simulink model "Test"  (R2018b)
settings: Solver=VariableStepAuto  StartTime=0.0  StopTime=10.0  RelTol=1e-3
undefined symbols (not defined in the file or in its folder): ExpectedOutputs, Inputs, sigbuilder_block, TestCase, TestInps, TestIters
libraries: fillib x3, library x2
(part 1 of 7)
settings Model: Creator=gauthamsm  LastModifiedBy=gauthamsm

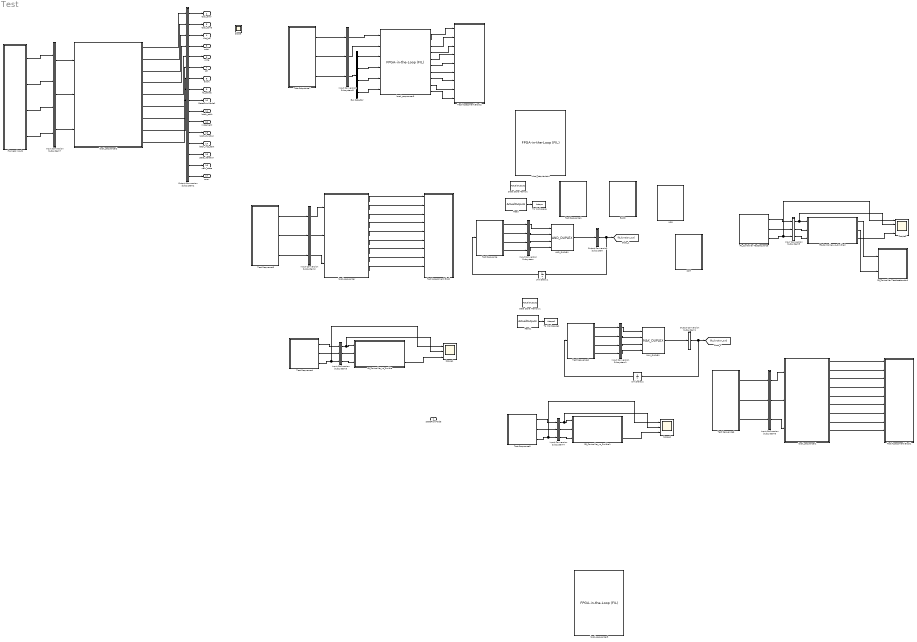
== system Test ==
  " XOR" : Test Sequence  TreatAsAtomicUnit=on
  AND_DUPLEX : library/AND_DUPLEX  SystemSampleTime=-1  VariantControl=MUX_FB
  BAND : Test Sequence  TreatAsAtomicUnit=on
  Bus Selector : BusSelector  OutputSignals=done,busy,error,code
  Data Store Memory : DataStoreMemory  DataStoreName=ActualOutputs  ReadBeforeWriteMsg=warning  WriteAfterWriteMsg=warning  WriteAfterReadMsg=warning  ShowAdditionalParam=off  OutDataTypeStr=int32  Dimensions=[TestIters, 3]
  Data Store Memory1 : DataStoreMemory  DataStoreName=ActualOutputs  ReadBeforeWriteMsg=warning  WriteAfterWriteMsg=warning  WriteAfterReadMsg=warning  ShowAdditionalParam=off  OutDataTypeStr=int32  Dimensions=[TestIters, 3]
  FB_Controller_vs_Smitha : ModelReference  ModelNameDialog=FB_Controller_vs_Smitha  SimulationMode=Normal  ModelReferenceVersion=1.41
  FB_Controller_vs_Smitha1 : ModelReference  ModelNameDialog=FB_Controller_vs_Smitha  SimulationMode=Normal  ModelReferenceVersion=1.41
  FB_Controller_vs_Smitha2 : ModelReference  ModelNameDialog=FB_Controller  SimulationMode=Normal  ModelReferenceVersion=1.46
  Fb_Controller TestAssessment : Test Sequence  TreatAsAtomicUnit=on
  Fb_Controller TestSequence : Test Sequence  TreatAsAtomicUnit=on
  Harness Inputs : Subsystem  Tag=STV Subsys  LoadFcn=sigbuilder_block('load');  StartFcn=sigbuilder_block('start');  StopFcn=sigbuilder_block('stop');  ClipboardFcn=sigbuilder_block('clipboard');  mask(Sigbuilder block){tuvar=[0:10]}
      mask init:
      | if ~strcmp(get_param(bdroot(gcb),'SimulationStatus'),'stopped'),tuvar = sigbuilder_block('maskInit'); end
      settings: CopyFcn=sigbuilder_block('copy');  DeleteFcn=sigbuilder_block('delete');  ModelCloseFcn=sigbuilder_block('modelClose');  PreSaveFcn=sigbuilder_block('preSave');  PauseFcn=sigbuilder_block('pause');  ContinueFcn=sigbuilder_block('continue');  NameChangeFcn=sigbuilder_block('namechange');  OpenFcn=sigbuilder_block('open',[5.4 30 1141.2 522.6 ]);  CloseFcn=sigbuilder_block('close');
      mask Display: plot(0, 0, 100, 100,[2, 2, 32, 32, 2], [68, 8, 8, 68, 68],[32, 2], [38, 38], [32, 19, 2],[53, 60, 44], [32, 17, 17, 2],[16, 16, 31, 31]);txt = getActiveGroup(gcbh);text(2, 100, txt,'verticalAlignment', 'top');
  Input Conversion Subsystem : Subsystem  Tag=__SLT_ICS__  Description=|
      | Signal spec.
      | and routing
      settings: AttributesFormatString=%<Description>
  Input Conversion Subsystem1 : Subsystem  Tag=__SLT_ICS__  Description=|
      | Signal spec.
      | and routing
      settings: AttributesFormatString=%<Description>
  Input Conversion Subsystem2 : Subsystem  Tag=__SLT_ICS__  Description=|
      | Signal spec.
      | and routing
      settings: AttributesFormatString=%<Description>
  Input Conversion Subsystem3 : Subsystem  Tag=__SLT_ICS__  Description=|
      | Signal spec.
      | and routing
      settings: AttributesFormatString=%<Description>
  Input Conversion Subsystem4 : Subsystem  Tag=__SLT_ICS__  Description=|
      | Signal spec.
      | and routing
      settings: AttributesFormatString=%<Description>
  Input Conversion Subsystem5 : Subsystem  Tag=__SLT_ICS__  Description=|
      | Signal spec.
      | and routing
      settings: AttributesFormatString=%<Description>
  Input Conversion Subsystem6 : Subsystem  Tag=__SLT_ICS__  Description=|
      | Signal spec.
      | and routing
      settings: AttributesFormatString=%<Description>
  Input Conversion Subsystem7 : Subsystem  Tag=__SLT_ICS__  Description=|
      | Signal spec.
      | and routing
      settings: AttributesFormatString=%<Description>
  Input Conversion Subsystem8 : Subsystem  Tag=__SLT_ICS__  Description=|
      | Signal spec.
      | and routing
      settings: AttributesFormatString=%<Description>
  MAX_DUPLEX : library/MAX_DUPLEX  SystemSampleTime=-1  VariantControl=MUX_FB
  NOT : Test Sequence  TreatAsAtomicUnit=on
  Output Conversion Subsystem : Subsystem  Tag=__SLT_OCS__  Description=|
      | Signal spec.
      | and routing
      settings: AttributesFormatString=%<Description>
  Output Conversion Subsystem1 : Subsystem  Tag=__SLT_OCS__  Description=|
      | Signal spec.
      | and routing
      settings: AttributesFormatString=%<Description>
  Output Conversion Subsystem2 : Subsystem  Tag=__SLT_OCS__  Description=|
      | Signal spec.
      | and routing
      settings: AttributesFormatString=%<Description>
  Read : DataStoreRead  DataStoreName=ActualOutputs
  Read1 : DataStoreRead  DataStoreName=ActualOutputs
  Scope : Scope
  Scope1 : Scope  NumInputPorts=3
  Scope2 : Scope  NumInputPorts=3
  Scope3 : Scope  NumInputPorts=4
  Test Assessment Block : Test Sequence  Tag=__SLT_ASMT__  TreatAsAtomicUnit=on
  Test Assessment Block1 : Test Sequence  Tag=__SLT_ASMT__  TreatAsAtomicUnit=on
  Test Assessment Block2 : Test Sequence  Tag=__SLT_ASMT__  TreatAsAtomicUnit=on
  Test Sequence : Test Sequence  TreatAsAtomicUnit=on
  Test Sequence1 : Test Sequence  TreatAsAtomicUnit=on
  Test Sequence2 : Test Sequence  TreatAsAtomicUnit=on
  Test Sequence3 : Test Sequence  TreatAsAtomicUnit=on
  Test Sequence4 : Test Sequence  TreatAsAtomicUnit=on
  Test Sequence5 : Test Sequence  TreatAsAtomicUnit=on
  Test Sequence6 : Test Sequence  TreatAsAtomicUnit=on
  Test Sequence7 : Test Sequence  TreatAsAtomicUnit=on
  To Workspace : ToWorkspace  VariableName=Actops  SampleTime=-1
  To Workspace1 : ToWorkspace  VariableName=Actops1  SampleTime=-1
  Unit Delay1 : UnitDelay  SampleTime=-1
  Unit Delay2 : UnitDelay  SampleTime=-1
  local_sequencer : ModelReference  ModelNameDialog=local_sequencer  SimulationMode=Normal  ModelReferenceVersion=1.256
  local_sequencer1 : ModelReference  ModelNameDialog=local_sequencer  SimulationMode=Normal  ModelReferenceVersion=1.256
  local_sequencer2 : ModelReference  ModelNameDialog=local_sequencer  SimulationMode=Normal  ModelReferenceVersion=1.256
  local_sequencer3 : fillib/FPGA-in-the-Loop (FIL)  ForceInterfaceUpdate=0.81472
  local_sequencer4 : fillib/FPGA-in-the-Loop (FIL)  ForceInterfaceUpdate=0.90579
  local_sequencer5 : fillib/FPGA-in-the-Loop (FIL)  ForceInterfaceUpdate=0.91338
  StateFlowMode : Outport
  task_error : Outport  Port=2  OutDataTypeStr=boolean  PortDimensions=[1]
  task_done : Outport  Port=3  OutDataTypeStr=boolean  PortDimensions=[1]
  inst_ptr : Outport  Port=4  OutDataTypeStr=uint32  PortDimensions=[1]
  addr : Outport  Port=5  OutDataTypeStr=fixdt('ufix8_En1000')  PortDimensions=[1]
  write : Outport  Port=6  OutDataTypeStr=boolean  PortDimensions=[1]
  ctrl : Outport  Port=7  OutDataTypeStr=boolean  PortDimensions=[1]
  abort : Outport  Port=8  OutDataTypeStr=boolean  PortDimensions=[1]
  fb_select : Outport  Port=9  OutDataTypeStr=uint8  PortDimensions=[1]
  StateFlowMode1 : Outport  Port=10  OutDataTypeStr=Enum: StateFlowModeType  PortDimensions=[1]
  latch_addr : Outport  Port=11  OutDataTypeStr=boolean  PortDimensions=[1]
  increment : Outport  Port=12  OutDataTypeStr=boolean  PortDimensions=[1]
  latch_function : Outport  Port=13  OutDataTypeStr=boolean  PortDimensions=[1]
  latch_inst_start : Outport  Port=14  OutDataTypeStr=boolean  PortDimensions=[1]
  state_iteration : Outport  Port=15  OutDataTypeStr=boolean  PortDimensions=[1]
  new_state : Outport  Port=16  OutDataTypeStr=boolean  PortDimensions=[1]
  error : Outport  Port=17  OutDataTypeStr=boolean  PortDimensions=[1]
  wires:
  Unit Delay1/1 -> Test Sequence/1(fb_functions_out)
  Output Conversion Subsystem/1(Outport_1) -> Unit Delay1/1, [fb_function_out]
  Input Conversion Subsystem/3(Outport_3) -> AND_DUPLEX/3
  AND_DUPLEX/1 -> Output Conversion Subsystem/1(Inport_1)
  Input Conversion Subsystem/4(Outport_4) -> AND_DUPLEX/4
  Test Sequence/2(fb_control) -> Input Conversion Subsystem/2(Inport_2)
  Input Conversion Subsystem/1(Outport_1) -> AND_DUPLEX/1
  Input Conversion Subsystem/2(Outport_2) -> AND_DUPLEX/2
  Test Sequence/3(dataInA) -> Input Conversion Subsystem/3(Inport_3)
  Test Sequence/4(dataInB) -> Input Conversion Subsystem/4(Inport_4)
  Test Sequence/1(fb_select) -> Input Conversion Subsystem/1(Inport_1)
  Read/1 -> To Workspace/1
  Input Conversion Subsystem1/3(Outport_3) -> MAX_DUPLEX/3
  Test Sequence2/4(dataInB) -> Input Conversion Subsystem1/4(Inport_4)
  Input Conversion Subsystem1/4(Outport_4) -> MAX_DUPLEX/4
  Unit Delay2/1 -> Test Sequence2/1(fb_functions_out)
  Output Conversion Subsystem1/1(Outport_1) -> Unit Delay2/1, [fb_function_out]
  Read1/1 -> To Workspace1/1
  Test Sequence2/1(fb_select) -> Input Conversion Subsystem1/1(Inport_1)
  Input Conversion Subsystem1/1(Outport_1) -> MAX_DUPLEX/1
  Input Conversion Subsystem1/2(Outport_2) -> MAX_DUPLEX/2
  MAX_DUPLEX/1 -> Output Conversion Subsystem1/1(Inport_1)
  Test Sequence2/2(fb_control) -> Input Conversion Subsystem1/2(Inport_2)
  Test Sequence2/3(dataInA) -> Input Conversion Subsystem1/3(Inport_3)
  Test Sequence3/2(inst) -> Input Conversion Subsystem2/2(Inport_2)
  local_sequencer/2 -> Test Assessment Block/2(task_done)  "task_done"
  local_sequencer/8 -> Test Assessment Block/8(fb_select)  "fb_select"
  ? -> Test Assessment Block/10(latch_addr)  "latch_addr"
  Input Conversion Subsystem2/1(Outport_1) -> local_sequencer/1
  Test Sequence3/1(trigger) -> Input Conversion Subsystem2/1(Inport_1)
  local_sequencer/3 -> Test Assessment Block/3(inst_ptr)  "inst_ptr"
  Input Conversion Subsystem2/3(Outport_3) -> local_sequencer/3
  Input Conversion Subsystem2/2(Outport_2) -> local_sequencer/2
  local_sequencer/1 -> Test Assessment Block/1(task_error)  "task_error"
  local_sequencer/7 -> Test Assessment Block/7(abort)  "abort"
  local_sequencer/6 -> Test Assessment Block/6(ctrl)  "ctrl"
  local_sequencer/9 -> Test Assessment Block/9(StateFlowMode)  "StateFlowMode"
  local_sequencer/5 -> Test Assessment Block/5(write)  "write"
  local_sequencer/4 -> Test Assessment Block/4(addr)  "addr"
  Test Sequence3/3(status) -> Input Conversion Subsystem2/3(Inport_3)
  Test Sequence4/3(fb_func_signals) -> Scope1/1, Input Conversion Subsystem3/3(Inport_3)
  Input Conversion Subsystem3/3(Outport_3) -> FB_Controller_vs_Smitha/3
  Test Sequence4/1(ctrl) -> Input Conversion Subsystem3/1(Inport_1)
  Input Conversion Subsystem3/1(Outport_1) -> Scope1/2, FB_Controller_vs_Smitha/1
  Test Sequence4/2(abort) -> Input Conversion Subsystem3/2(Inport_2)
  FB_Controller_vs_Smitha/3 -> Scope1/3
  Input Conversion Subsystem3/2(Outport_2) -> FB_Controller_vs_Smitha/2
  FB_Controller_vs_Smitha1/3 -> Scope2/3
  Input Conversion Subsystem4/1(Outport_1) -> Scope2/2, FB_Controller_vs_Smitha1/1
  Input Conversion Subsystem4/2(Outport_2) -> FB_Controller_vs_Smitha1/2
  Input Conversion Subsystem4/3(Outport_3) -> FB_Controller_vs_Smitha1/3
  Test Sequence5/3(fb_func_signals) -> Scope2/1, Input Conversion Subsystem4/3(Inport_3)
  Test Sequence5/2(abort) -> Input Conversion Subsystem4/2(Inport_2)
  Test Sequence5/1(ctrl) -> Input Conversion Subsystem4/1(Inport_1)
  Fb_Controller TestSequence/3(fb_func_signals) -> Scope3/1, Input Conversion Subsystem5/3(Inport_3)
  Fb_Controller TestSequence/2(abort) -> Input Conversion Subsystem5/2(Inport_2)
  Input Conversion Subsystem5/2(Outport_2) -> FB_Controller_vs_Smitha2/2
  FB_Controller_vs_Smitha2/3 -> Scope3/4
  FB_Controller_vs_Smitha2/2 -> Fb_Controller TestAssessment/2(status)
  FB_Controller_vs_Smitha2/1 -> Fb_Controller TestAssessment/1(fb_control)
  Fb_Controller TestSequence/1(ctrl) -> Input Conversion Subsystem5/1(Inport_1)
  Input Conversion Subsystem5/1(Outport_1) -> Scope3/2, FB_Controller_vs_Smitha2/1
  Input Conversion Subsystem5/3(Outport_3) -> FB_Controller_vs_Smitha2/3
  local_sequencer1/5 -> Test Assessment Block1/5(write)  "write"
  ? -> Test Assessment Block1/10(latch_addr)  "latch_addr"
  local_sequencer1/9 -> Test Assessment Block1/9(StateFlowMode)  "StateFlowMode"
  local_sequencer1/6 -> Test Assessment Block1/6(ctrl)  "ctrl"
  local_sequencer1/7 -> Test Assessment Block1/7(abort)  "abort"
  local_sequencer1/8 -> Test Assessment Block1/8(fb_select)  "fb_select"
  local_sequencer1/3 -> Test Assessment Block1/3(inst_ptr)  "inst_ptr"
  Test Sequence6/1(trigger) -> Input Conversion Subsystem6/1(Inport_1)
  local_sequencer1/4 -> Test Assessment Block1/4(addr)  "addr"
  Test Sequence6/2(inst) -> Input Conversion Subsystem6/2(Inport_2)
  local_sequencer1/1 -> Test Assessment Block1/1(task_error)  "task_error"
  local_sequencer1/2 -> Test Assessment Block1/2(task_done)  "task_done"
  Input Conversion Subsystem6/3(Outport_3) -> local_sequencer1/3
  Test Sequence6/3(status) -> Input Conversion Subsystem6/3(Inport_3)
  Input Conversion Subsystem6/2(Outport_2) -> local_sequencer1/2
  Input Conversion Subsystem6/1(Outport_1) -> local_sequencer1/1
  Output Conversion Subsystem2/6(Outport_6) -> ctrl/1
  Output Conversion Subsystem2/3(Outport_3) -> inst_ptr/1
  ? -> Output Conversion Subsystem2/13(Inport_13)
  local_sequencer2/5 -> Output Conversion Subsystem2/5(Inport_5)
  local_sequencer2/9 -> Output Conversion Subsystem2/9(Inport_9)
  Input Conversion Subsystem7/3(Outport_3) -> local_sequencer2/3
  Output Conversion Subsystem2/16(Outport_16) -> error/1
  ? -> Output Conversion Subsystem2/10(Inport_10)
  Input Conversion Subsystem7/1(Outport_1) -> local_sequencer2/1
  local_sequencer2/7 -> Output Conversion Subsystem2/7(Inport_7)
  Output Conversion Subsystem2/13(Outport_13) -> latch_inst_start/1
  local_sequencer2/6 -> Output Conversion Subsystem2/6(Inport_6)
  Output Conversion Subsystem2/9(Outport_9) -> StateFlowMode1/1
  Output Conversion Subsystem2/11(Outport_11) -> increment/1
  local_sequencer2/3 -> Output Conversion Subsystem2/3(Inport_3)
  local_sequencer2/1 -> Output Conversion Subsystem2/1(Inport_1)
  Output Conversion Subsystem2/14(Outport_14) -> state_iteration/1
  local_sequencer2/8 -> Output Conversion Subsystem2/8(Inport_8)
  Output Conversion Subsystem2/15(Outport_15) -> new_state/1
  Input Conversion Subsystem7/2(Outport_2) -> local_sequencer2/2
  local_sequencer2/2 -> Output Conversion Subsystem2/2(Inport_2)
  Harness Inputs/4(status.code) -> Input Conversion Subsystem7/4(Inport_4)
  ? -> Output Conversion Subsystem2/14(Inport_14)
  Output Conversion Subsystem2/5(Outport_5) -> write/1
  local_sequencer2/4 -> Output Conversion Subsystem2/4(Inport_4)
  ? -> Output Conversion Subsystem2/16(Inport_16)
  Harness Inputs/2(inst) -> Input Conversion Subsystem7/2(Inport_2)
  Output Conversion Subsystem2/2(Outport_2) -> task_done/1
  ? -> Output Conversion Subsystem2/12(Inport_12)
  Output Conversion Subsystem2/1(Outport_1) -> task_error/1
  Output Conversion Subsystem2/8(Outport_8) -> fb_select/1
  Harness Inputs/1(trigger) -> Input Conversion Subsystem7/1(Inport_1)
  Output Conversion Subsystem2/7(Outport_7) -> abort/1
  Output Conversion Subsystem2/10(Outport_10) -> latch_addr/1
  Output Conversion Subsystem2/12(Outport_12) -> latch_function/1
  ? -> Output Conversion Subsystem2/15(Inport_15)
  Harness Inputs/3(status.error) -> Input Conversion Subsystem7/3(Inport_3)
  ? -> Output Conversion Subsystem2/11(Inport_11)
  Output Conversion Subsystem2/4(Outport_4) -> addr/1
  Bus Selector/4 -> local_sequencer5/6  "<code>"
  Test Sequence7/3(status) -> Input Conversion Subsystem8/3(Inport_3)
  Test Sequence7/1(trigger) -> Input Conversion Subsystem8/1(Inport_1)
  Input Conversion Subsystem8/1(Outport_1) -> local_sequencer5/1
  Test Sequence7/2(inst) -> Input Conversion Subsystem8/2(Inport_2)
  local_sequencer5/10 -> Test Assessment Block2/9(latch_addr)
  Bus Selector/2 -> local_sequencer5/4  "<busy>"
  local_sequencer5/5 -> Test Assessment Block2/4(addr)
  local_sequencer5/8 -> Test Assessment Block2/7(abort)
  local_sequencer5/3 -> Test Assessment Block2/2(task_done)
  local_sequencer5/6 -> Test Assessment Block2/5(write)
  local_sequencer5/2 -> Test Assessment Block2/1(task_error)
  local_sequencer5/4 -> Test Assessment Block2/3(inst_ptr)
  Input Conversion Subsystem8/2(Outport_2) -> local_sequencer5/2
  Bus Selector/1 -> local_sequencer5/3  "<done>"
  local_sequencer5/7 -> Test Assessment Block2/6(ctrl)
  Bus Selector/3 -> local_sequencer5/5  "<error>"
  Input Conversion Subsystem8/3(Outport_3) -> Bus Selector/1
  local_sequencer5/9 -> Test Assessment Block2/8(fb_select)

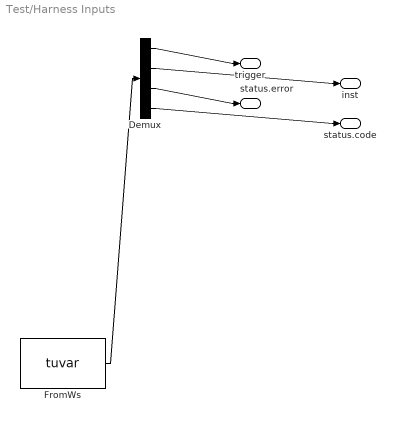
== system Test/Harness Inputs ==
  Demux : Demux  Tag=STV Demux
  FromWs : FromWorkspace  Tag=STV FromWs  VariableName=tuvar  SampleTime=0
      SigBuilderData=|
      | dataSet(1).timeRange = [0 6]
      | dataSet(1).name = 'Test Case 1'
      | dataSet(2).timeRange = [0 7]
      | dataSet(2).name = 'Test Case 2'
      | dataSet(3).timeRange = [0 8]
      | dataSet(3).name = 'Test Case 3'
      | dataSet(4).timeRange = [0 9]
      | dataSet(4).name = 'Test Case 4'
      | dataSet(5).timeRange = [0 10]
      | dataSet(5).name = 'Test Case 5'
      | dataSet(6).timeRange = [0 12]
      | dataSet(6).name = 'Test Case 6'
      | dataSet(7).timeRange = [0 14]
      | dataSet(7).name = 'Test Case 7'
      | dataSet(8).timeRange = [0 15]
      | dataSet(8).name = 'Test Case 8'
      | dataSet(9).timeRange = [0 16]
      | dataSet(9).name = 'Test Case 9'
      | dataSet(10).timeRange = [0 17]
      | dataSet(10).name = 'Test Case 10'
      | dataSet(11).timeRange = [0 18]
      | dataSet(11).name = 'Test Case 11'
      | sbobj.Name = 'Signal Builder'
      | sbobj.Groups(1).Name = 'Test Case 1'
      | sbobj.Groups(1).Signals(1).Name = 'trigger'
      | sbobj.Groups(1).Signals(1).XData = [0 1 1 2 3 4 5 6]
      | sbobj.Groups(1).Signals(1).YData = [1 1 0 0 0 0 0 0]
      | sbobj.Groups(1).Signals(2).Name = 'inst'
      | sbobj.Groups(1).Signals(2).XData = [0 1 2 3 4 5 6]
      | sbobj.Groups(1).Signals(2).YData = [2147483646 2147483646 2147483646 2147483646 2147483646 2147483646 2147483646]
      | sbobj.Groups(1).Signals(3).Name = 'status.error'
      | sbobj.Groups(1).Signals(3).XData = [0 1 2 3 3 4 5 5 6]
      | sbobj.Groups(1).Signals(3).YData = [1 1 1 1 0 0 0 1 1]
      | sbobj.Groups(1).Signals(4).Name = 'status.code'
      | sbobj.Groups(1).Signals(4).XData = [0 1 1 2 2 3 3 4 4 5 5 6]
      | sbobj.Groups(1).Signals(4).YData = [2151677953 2151677953 1 1 268435457 268435457 1 1 255852545 255852545 268435457 268435457]
      | sbobj.Groups(1).TimeRange = [0 6]
      | sbobj.Groups(2).Name = 'Test Case 2'
      | sbobj.Groups(2).Signals(1).Name = 'trigger'
      | sbobj.Groups(2).Signals(1).XData = [0 1 1 2 2 3 3 5 5 6 6 7]
      | sbobj.Groups(2).Signals(1).YData = [1 1 0 0 0 0 0 0 0 0 0 0]
      | sbobj.Groups(2).Signals(2).Name = 'inst'
      | sbobj.Groups(2).Signals(2).XData = [0 1 1 2 2 3 3 5 5 6 6 7]
      | sbobj.Groups(2).Signals(2).YData = [2147483646 2147483646 2147483646 2147483646 2147483646 2147483646 2147483646 2147483646 2147483646 2147483646 2147483646 2147483646]
      | sbobj.Groups(2).Signals(3).Name = 'status.error'
      | sbobj.Groups(2).Signals(3).XData = [0 1 1 2 2 3 3 5 5 6 6 7]
      | sbobj.Groups(2).Signals(3).YData = [1 1 1 1 1 1 0 0 0 0 1 1]
      | sbobj.Groups(2).Signals(4).Name = 'status.code'
      | sbobj.Groups(2).Signals(4).XData = [0 1 1 2 2 3 3 5 5 6 6 7]
      | sbobj.Groups(2).Signals(4).YData = [2151677953 2151677953 1 1 268435457 268435457 1 1 524288001 524288001 528482305 528482305]
      | sbobj.Groups(2).TimeRange = [0 7]
      | sbobj.Groups(3).Name = 'Test Case 3'
      | sbobj.Groups(3).Signals(1).Name = 'trigger'
      | sbobj.Groups(3).Signals(1).XData = [0 1 1 2 2 3 3 6 6 7 7 8]
      | sbobj.Groups(3).Signals(1).YData = [1 1 0 0 0 0 0 0 0 0 0 0]
      | sbobj.Groups(3).Signals(2).Name = 'inst'
      | sbobj.Groups(3).Signals(2).XData = [0 1 1 2 2 3 3 6 6 7 7 8]
      | sbobj.Groups(3).Signals(2).YData = [2147483646 2147483646 2147483646 2147483646 2147483646 2147483646 2147483646 2147483646 2147483646 2147483646 2147483646 2147483646]
      | sbobj.Groups(3).Signals(3).Name = 'status.error'
      | sbobj.Groups(3).Signals(3).XData = [0 1 1 2 2 3 3 6 6 7 7 8]
      | sbobj.Groups(3).Signals(3).YData = [1 1 1 1 1 1 0 0 0 0 1 1]
      | sbobj.Groups(3).Signals(4).Name = 'status.code'
      | sbobj.Groups(3).Signals(4).XData = [0 1 1 2 2 3 3 6 6 7 7 8]
      | sbobj.Groups(3).Signals(4).YData = [2151677953 2151677953 1 1 268435457 268435457 1 1 255852545 255852545 260046849 260046849]
      | sbobj.Groups(3).TimeRange = [0 8]
      | sbobj.Groups(4).Name = 'Test Case 4'
      | sbobj.Groups(4).Signals(1).Name = 'trigger'
      | sbobj.Groups(4).Signals(1).XData = [0 1 1 2 2 3 3 5 5 7 7 8 8 9]
      | sbobj.Groups(4).Signals(1).YData = [1 1 0 0 0 0 0 0 0 0 0 0 0 0]
      | sbobj.Groups(4).Signals(2).Name = 'inst'
      | sbobj.Groups(4).Signals(2).XData = [0 1 1 2 2 3 3 5 5 7 7 8 8 9]
      | sbobj.Groups(4).Signals(2).YData = [2147483646 2147483646 2147483646 2147483646 2147483646 2147483646 2147483646 2147483646 2147483646 2147483646 2147483646 2147483646 2147483646 2147483646]
      | sbobj.Groups(4).Signals(3).Name = 'status.error'
      | sbobj.Groups(4).Signals(3).XData = [0 1 1 2 2 3 3 5 5 7 7 8 8 9]
      | sbobj.Groups(4).Signals(3).YData = [1 1 1 1 1 1 0 0 0 0 0 0 1 1]
      | sbobj.Groups(4).Signals(4).Name = 'status.code'
      | sbobj.Groups(4).Signals(4).XData = [0 1 1 2 2 3 3 5 5 7 7 8 8 9]
      | sbobj.Groups(4).Signals(4).YData = [2151677953 2151677953 1 1 268435457 268435457 1 1 268435457 268435457 524288001 524288001 528482305 528482305]
      | sbobj.Groups(4).TimeRange = [0 9]
      | sbobj.Groups(5).Name = 'Test Case 5'
      | sbobj.Groups(5).Signals(1).Name = 'trigger'
      | sbobj.Groups(5).Signals(1).XData = [0 1 1 2 2 3 3 5 5 8 8 9 9 10]
      | sbobj.Groups(5).Signals(1).YData = [1 1 0 0 0 0 0 0 0 0 0 0 0 0]
      | sbobj.Groups(5).Signals(2).Name = 'inst'
      | sbobj.Groups(5).Signals(2).XData = [0 1 1 2 2 3 3 5 5 8 8 9 9 10]
      | sbobj.Groups(5).Signals(2).YData = [2147483646 2147483646 2147483646 2147483646 2147483646 2147483646 2147483646 2147483646 2147483646 2147483646 2147483646 2147483646 2147483646 2147483646]
      | sbobj.Groups(5).Signals(3).Name = 'status.error'
      | sbobj.Groups(5).Signals(3).XData = [0 1 1 2 2 3 3 5 5 8 8 9 9 10]
      | sbobj.Groups(5).Signals(3).YData = [1 1 1 1 1 1 0 0 0 0 0 0 1 1]
      | sbobj.Groups(5).Signals(4).Name = 'status.code'
      | sbobj.Groups(5).Signals(4).XData = [0 1 1 2 2 3 3 5 5 8 8 9 9 10]
      | sbobj.Groups(5).Signals(4).YData = [2151677953 2151677953 2428502017 2428502017 268435457 268435457 1 1 268435457 268435457 524288001 524288001 528482305 528482305]
      | sbobj.Groups(6).Name = 'Test Case 6'
      | sbobj.Groups(6).Signals(1).Name = 'trigger'
      | sbobj.Groups(6).Signals(1).XData = [0 1 1 2 2 3 3 5 5 7 7 8 8 9 9 10 10 11 11 12]
      | sbobj.Groups(6).Signals(1).YData = [1 1 0 0 0 0 0 0 0 0 0 0 0 0 0 0 0 0 0 0]
      | sbobj.Groups(6).Signals(2).Name = 'inst'
      | sbobj.Groups(6).Signals(2).XData = [0 1 1 2 2 3 3 5 5 7 7 8 8 9 9 10 10 11 11 12]
      | sbobj.Groups(6).Signals(2).YData = [2147483646 2147483646 2147483646 2147483646 2147483646 2147483646 2147483646 2147483646 2147483646 2147483646 2147483646 2147483646 2147483646 2147483646 2147483646 2147483646 2147483646 2147483646 2147483646 2147483646]
      | sbobj.Groups(6).Signals(3).Name = 'status.error'
      | sbobj.Groups(6).Signals(3).XData = [0 1 1 2 2 3 3 5 5 7 7 8 8 9 9 10 10 11 11 12]
      | sbobj.Groups(6).Signals(3).YData = [1 1 1 1 1 1 0 0 0 0 0 0 0 0 0 0 0 0 1 1]
      | sbobj.Groups(6).Signals(4).Name = 'status.code'
      | sbobj.Groups(6).Signals(4).XData = [0 1 1 2 2 3 3 5 5 7 7 8 8 9 9 10 10 11 11 12]
      | sbobj.Groups(6).Signals(4).YData = [2160066561 2160066561 1 1 268435457 268435457 1 1 268435457 268435457 1 1 4194305 4194305 268435457 268435457 524288001 524288001 268435457 268435457]
      | sbobj.Groups(6).TimeRange = [0 12]
      | sbobj.Groups(7).Name = 'Test Case 7'
      | sbobj.Groups(7).Signals(1).Name = 'trigger'
      | sbobj.Groups(7).Signals(1).XData = [0 1 1 2 2 3 3 5 5 9 9 11 11 12 12 13 13 14]
      | sbobj.Groups(7).Signals(1).YData = [1 1 0 0 0 0 0 0 0 0 0 0 0 0 0 0 0 0]
      | sbobj.Groups(7).Signals(2).Name = 'inst'
      | sbobj.Groups(7).Signals(2).XData = [0 1 1 2 2 3 3 5 5 9 9 11 11 12 12 13 13 14]
      | sbobj.Groups(7).Signals(2).YData = [2147483646 2147483646 2147483646 2147483646 2147483646 2147483646 2147483646 2147483646 2147483646 2147483646 2147483646 2147483646 2147483646 2147483646 2147483646 2147483646 2147483646 2147483646]
      | sbobj.Groups(7).Signals(3).Name = 'status.error'
      | sbobj.Groups(7).Signals(3).XData = [0 1 1 2 2 3 3 5 5 9 9 11 11 12 12 13 13 14]
      | sbobj.Groups(7).Signals(3).YData = [1 1 1 1 1 1 0 0 0 0 0 0 0 0 0 0 1 1]
      | sbobj.Groups(7).Signals(4).Name = 'status.code'
      | sbobj.Groups(7).Signals(4).XData = [0 1 1 2 2 3 3 5 5 9 9 11 11 12 12 13 13 14]
      | sbobj.Groups(7).Signals(4).YData = [2151677953 2151677953 1 1 268435457 268435457 1 1 268435457 268435457 1 1 268435457 268435457 255852545 255852545 1 1]
      | sbobj.Groups(7).TimeRange = [0 14]
      | sbobj.Groups(8).Name = 'Test Case 8'
      | sbobj.Groups(8).Signals(1).Name = 'trigger'
      | sbobj.Groups(8).Signals(1).XData = [0 1 1 2 2 3 3 5 5 9 9 11 11 12 12 13 13 14 14 15]
      | sbobj.Groups(8).Signals(1).YData = [1 1 0 0 0 0 0 0 0 0 0 0 0 0 0 0 0 0 0 0]
      | sbobj.Groups(8).Signals(2).Name = 'inst'
      | sbobj.Groups(8).Signals(2).XData = [0 1 1 2 2 3 3 5 5 9 9 11 11 12 12 13 13 14 14 15]
      | sbobj.Groups(8).Signals(2).YData = [2147483646 2147483646 2147483646 2147483646 2147483646 2147483646 2147483646 2147483646 2147483646 2147483646 2147483646 2147483646 2147483646 2147483646 2147483646 2147483646 2147483646 2147483646 2147483646 2147483646]
      | sbobj.Groups(8).Signals(3).Name = 'status.error'
      | sbobj.Groups(8).Signals(3).XData = [0 1 1 2 2 3 3 5 5 9 9 11 11 12 12 13 13 14 14 15]
      | sbobj.Groups(8).Signals(3).YData = [1 1 1 1 1 1 0 0 0 0 0 0 0 0 0 0 0 0 1 1]
      | sbobj.Groups(8).Signals(4).Name = 'status.code'
      | sbobj.Groups(8).Signals(4).XData = [0 1 1 2 2 3 3 5 5 9 9 11 11 12 12 13 13 14 14 15]
      | sbobj.Groups(8).Signals(4).YData = [2151677953 2151677953 1 1 268435457 268435457 1 1 268435457 268435457 1 1 268435457 268435457 1 1 255852545 255852545 1 1]
      | sbobj.Groups(8).TimeRange = [0 15]
      | sbobj.Groups(9).Name = 'Test Case 9'
      | sbobj.Groups(9).Signals(1).Name = 'trigger'
      | sbobj.Groups(9).Signals(1).XData = [0 1 1 2 2 3 3 5 5 9 9 10 10 11 11 13 13 15 15 16]
      | sbobj.Groups(9).Signals(1).YData = [1 1 0 0 0 0 0 0 0 0 0 0 0 0 0 0 0 0 0 0]
      | sbobj.Groups(9).Signals(2).Name = 'inst'
      | sbobj.Groups(9).Signals(2).XData = [0 1 1 2 2 3 3 5 5 9 9 10 10 11 11 13 13 15 15 16]
      | sbobj.Groups(9).Signals(2).YData = [2147483646 2147483646 2147483646 2147483646 2147483646 2147483646 2147483646 2147483646 2147483646 2147483646 2147483646 2147483646 2147483646 2147483646 2147483646 2147483646 2147483646 2147483646 2147483646 2147483646]
      | sbobj.Groups(9).Signals(3).Name = 'status.error'
      | sbobj.Groups(9).Signals(3).XData = [0 1 1 2 2 3 3 5 5 9 9 10 10 11 11 13 13 15 15 16]
      | sbobj.Groups(9).Signals(3).YData = [1 1 1 1 1 1 0 0 0 0 0 0 0 0 0 0 0 0 1 1]
      | sbobj.Groups(9).Signals(4).Name = 'status.code'
      | sbobj.Groups(9).Signals(4).XData = [0 1 1 2 2 3 3 5 5 9 9 10 10 11 11 13 13 15 15 16]
      | sbobj.Groups(9).Signals(4).YData = [2151677953 2151677953 1 1 268435457 268435457 1 1 268435457 268435457 1 1 268435457 268435457 1 1 260046849 260046849 1 1]
      | sbobj.Groups(9).TimeRange = [0 16]
      | sbobj.Groups(10).Name = 'Test Case 10'
      | sbobj.Groups(10).Signals(1).Name = 'trigger'
      | sbobj.Groups(10).Signals(1).XData = [0 1 1 2 2 3 3 5 5 9 9 11 11 12 12 14 14 16 16 17]
      | sbobj.Groups(10).Signals(1).YData = [1 1 0 0 0 0 0 0 0 0 0 0 0 0 0 0 0 0 0 0]
      | sbobj.Groups(10).Signals(2).Name = 'inst'
      | sbobj.Groups(10).Signals(2).XData = [0 1 1 2 2 3 3 5 5 9 9 11 11 12 12 14 14 16 16 17]
      | sbobj.Groups(10).Signals(2).YData = [2147483646 2147483646 2147483646 2147483646 2147483646 2147483646 2147483646 2147483646 2147483646 2147483646 2147483646 2147483646 2147483646 2147483646 2147483646 2147483646 2147483646 2147483646 2147483646 2147483646]
      | sbobj.Groups(10).Signals(3).Name = 'status.error'
      | sbobj.Groups(10).Signals(3).XData = [0 1 1 2 2 3 3 5 5 9 9 11 11 12 12 14 14 16 16 17]
      | sbobj.Groups(10).Signals(3).YData = [1 1 1 1 1 1 0 0 0 0 0 0 0 0 0 0 0 0 1 1]
      | sbobj.Groups(10).Signals(4).Name = 'status.code'
      | sbobj.Groups(10).Signals(4).XData = [0 1 1 2 2 3 3 5 5 9 9 11 11 12 12 14 14 16 16 17]
      | sbobj.Groups(10).Signals(4).YData = [2147483649 2147483649 1 1 268435457 268435457 1 1 268435457 268435457 1 1 268435457 268435457 1 1 260046849 260046849 1 1]
      | sbobj.Groups(10).TimeRange = [0 17]
      | sbobj.Groups(11).Name = 'Test Case 11'
      | sbobj.Groups(11).Signals(1).Name = 'trigger'
      | sbobj.Groups(11).Signals(1).XData = [0 1 1 2 3 5 9 11 12 14 16 16 17 17 18]
      | sbobj.Groups(11).Signals(1).YData = [1 1 0 0 0 0 0 0 0 0 0 1 1 0 0]
      | sbobj.Groups(11).Signals(2).Name = 'inst'
      | sbobj.Groups(11).Signals(2).XData = [0 1 2 3 5 9 11 12 14 16 17 18]
      | sbobj.Groups(11).Signals(2).YData = [2147483646 2147483646 2147483646 2147483646 2147483646 2147483646 2147483646 2147483646 2147483646 2147483646 2147483646 2147483646]
      | sbobj.Groups(11).Signals(3).Name = 'status.error'
      | sbobj.Groups(11).Signals(3).XData = [0 1 2 3 3 5 9 11 12 14 16 17 17 18]
      | sbobj.Groups(11).Signals(3).YData = [1 1 1 1 0 0 0 0 0 0 0 0 1 1]
      | sbobj.Groups(11).Signals(4).Name = 'status.code'
      | sbobj.Groups(11).Signals(4).XData = [0 1 1 2 2 3 3 5 5 9 9 11 11 12 12 14 14 16 16 17 17 18]
      | sbobj.Groups(11).Signals(4).YData = [2151677953 2151677953 1 1 268435457 268435457 1 1 268435457 268435457 1 1 268435457 268435457 1 1 2407530497 2407530497 260046849 260046849 268435457 268435457]
      | sbobj.Groups(11).TimeRange = [0 18]
  trigger : Outport  Tag=STV Outport
  inst : Outport  Tag=STV Outport  Port=2
  status.error : Outport  Tag=STV Outport  Port=3
  status.code : Outport  Tag=STV Outport  Port=4
  wires:
  FromWs/1 -> Demux/1
  Demux/1 -> trigger/1
  Demux/2 -> inst/1
  Demux/3 -> status.error/1
  Demux/4 -> status.code/1

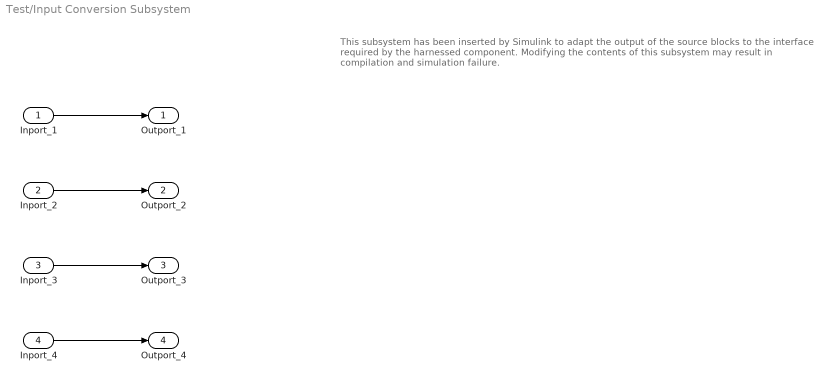
== system Test/Input Conversion Subsystem ==
  note: This subsystem has been inserted by Simulink to adapt the output of the source blocks to the interface required by the harnessed component.
      |  Modifying the contents of this subsystem may result in compilation and simulation failure.
  Inport_1 : Inport
  Inport_2 : Inport  Port=2
  Inport_3 : Inport  Port=3
  Inport_4 : Inport  Port=4
  Outport_1 : Outport
  Outport_2 : Outport  Port=2
  Outport_3 : Outport  Port=3
  Outport_4 : Outport  Port=4
  wires:
  Inport_1/1 -> Outport_1/1
  Inport_2/1 -> Outport_2/1
  Inport_3/1 -> Outport_3/1
  Inport_4/1 -> Outport_4/1

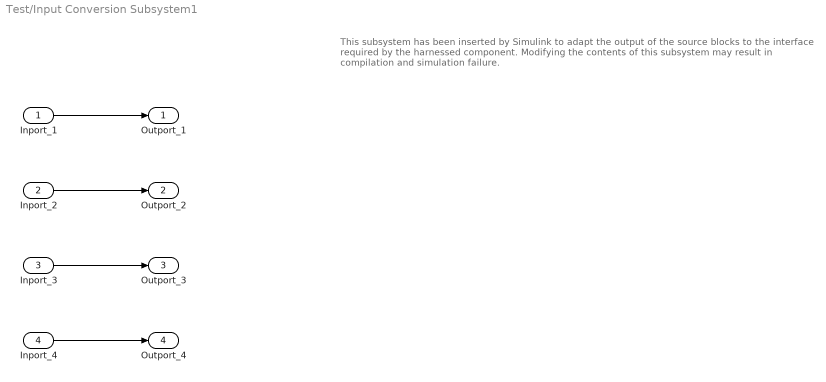
== system Test/Input Conversion Subsystem1 ==
  note: This subsystem has been inserted by Simulink to adapt the output of the source blocks to the interface required by the harnessed component.
      |  Modifying the contents of this subsystem may result in compilation and simulation failure.
  Inport_1 : Inport
  Inport_2 : Inport  Port=2
  Inport_3 : Inport  Port=3
  Inport_4 : Inport  Port=4
  Outport_1 : Outport
  Outport_2 : Outport  Port=2
  Outport_3 : Outport  Port=3
  Outport_4 : Outport  Port=4
  wires:
  Inport_1/1 -> Outport_1/1
  Inport_2/1 -> Outport_2/1
  Inport_3/1 -> Outport_3/1
  Inport_4/1 -> Outport_4/1

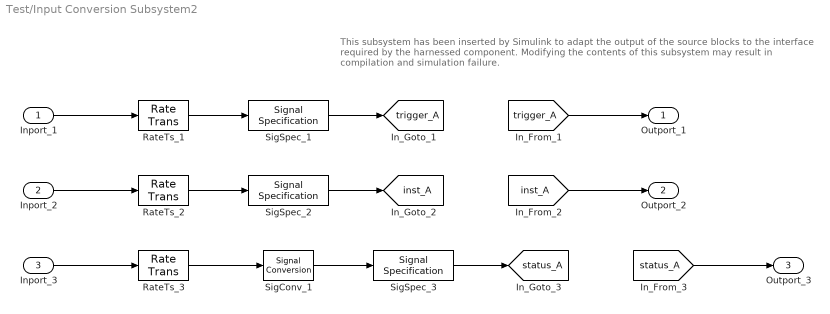
== system Test/Input Conversion Subsystem2 ==
  note: This subsystem has been inserted by Simulink to adapt the output of the source blocks to the interface required by the harnessed component.
      |  Modifying the contents of this subsystem may result in compilation and simulation failure.
  Inport_1 : Inport
  Inport_2 : Inport  Port=2
  Inport_3 : Inport  Port=3
  RateTs_1 : RateTransition  OutPortSampleTime=1
  RateTs_2 : RateTransition  OutPortSampleTime=1
  RateTs_3 : RateTransition  OutPortSampleTime=1
  SigConv_1 : SignalConversion  ConversionOutput=Virtual bus  OverrideOpt=off
  SigSpec_1 : SignalSpecification  OutDataTypeStr=boolean  Dimensions=[1]  SampleTime=1
  SigSpec_2 : SignalSpecification  OutDataTypeStr=int32  Dimensions=[1]  SampleTime=1
  SigSpec_3 : SignalSpecification  OutDataTypeStr=Bus: fb_status  SampleTime=1
  Outport_1 : Outport
  Outport_2 : Outport  Port=2
  Outport_3 : Outport  Port=3
  tag scope: inst_A=global, status_A=global, trigger_A=global
  wires:
  [trigger_A] -> Outport_1/1
  SigSpec_1/1 -> [trigger_A]
  RateTs_1/1 -> SigSpec_1/1
  Inport_1/1 -> RateTs_1/1
  [inst_A] -> Outport_2/1
  SigSpec_2/1 -> [inst_A]
  RateTs_2/1 -> SigSpec_2/1
  Inport_2/1 -> RateTs_2/1
  [status_A] -> Outport_3/1
  SigSpec_3/1 -> [status_A]
  SigConv_1/1 -> SigSpec_3/1
  RateTs_3/1 -> SigConv_1/1
  Inport_3/1 -> RateTs_3/1

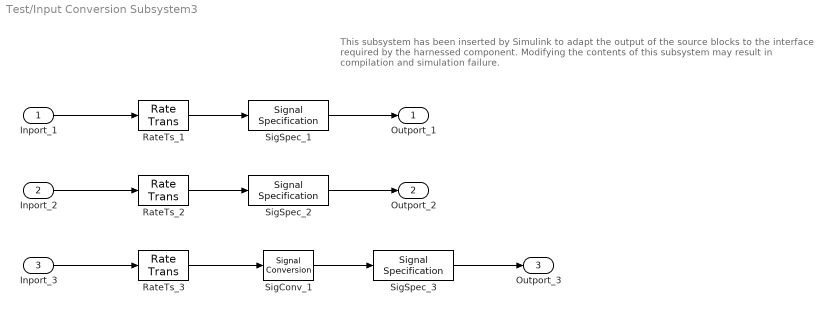
== system Test/Input Conversion Subsystem3 ==
  note: This subsystem has been inserted by Simulink to adapt the output of the source blocks to the interface required by the harnessed component.
      |  Modifying the contents of this subsystem may result in compilation and simulation failure.
  Inport_1 : Inport
  Inport_2 : Inport  Port=2
  Inport_3 : Inport  Port=3
  RateTs_1 : RateTransition  OutPortSampleTime=1
  RateTs_2 : RateTransition  OutPortSampleTime=1
  RateTs_3 : RateTransition  OutPortSampleTime=1
  SigConv_1 : SignalConversion  ConversionOutput=Virtual bus  OverrideOpt=off
  SigSpec_1 : SignalSpecification  OutDataTypeStr=boolean  Dimensions=[1]  SampleTime=1
  SigSpec_2 : SignalSpecification  OutDataTypeStr=boolean  Dimensions=[1]  SampleTime=1
  SigSpec_3 : SignalSpecification  OutDataTypeStr=Bus: fb_functions_out  SampleTime=1
  Outport_1 : Outport
  Outport_2 : Outport  Port=2
  Outport_3 : Outport  Port=3
  wires:
  SigSpec_1/1 -> Outport_1/1
  RateTs_1/1 -> SigSpec_1/1
  Inport_1/1 -> RateTs_1/1
  SigSpec_2/1 -> Outport_2/1
  RateTs_2/1 -> SigSpec_2/1
  Inport_2/1 -> RateTs_2/1
  SigSpec_3/1 -> Outport_3/1
  SigConv_1/1 -> SigSpec_3/1
  RateTs_3/1 -> SigConv_1/1
  Inport_3/1 -> RateTs_3/1

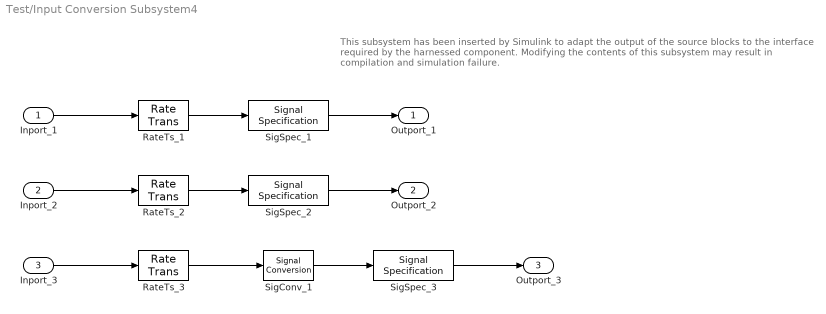
== system Test/Input Conversion Subsystem4 ==
  note: This subsystem has been inserted by Simulink to adapt the output of the source blocks to the interface required by the harnessed component.
      |  Modifying the contents of this subsystem may result in compilation and simulation failure.
  Inport_1 : Inport
  Inport_2 : Inport  Port=2
  Inport_3 : Inport  Port=3
  RateTs_1 : RateTransition  OutPortSampleTime=1
  RateTs_2 : RateTransition  OutPortSampleTime=1
  RateTs_3 : RateTransition  OutPortSampleTime=1
  SigConv_1 : SignalConversion  ConversionOutput=Virtual bus  OverrideOpt=off
  SigSpec_1 : SignalSpecification  OutDataTypeStr=boolean  Dimensions=[1]  SampleTime=1
  SigSpec_2 : SignalSpecification  OutDataTypeStr=boolean  Dimensions=[1]  SampleTime=1
  SigSpec_3 : SignalSpecification  OutDataTypeStr=Bus: fb_functions_out  SampleTime=1
  Outport_1 : Outport
  Outport_2 : Outport  Port=2
  Outport_3 : Outport  Port=3
  wires:
  SigSpec_1/1 -> Outport_1/1
  RateTs_1/1 -> SigSpec_1/1
  Inport_1/1 -> RateTs_1/1
  SigSpec_2/1 -> Outport_2/1
  RateTs_2/1 -> SigSpec_2/1
  Inport_2/1 -> RateTs_2/1
  SigSpec_3/1 -> Outport_3/1
  SigConv_1/1 -> SigSpec_3/1
  RateTs_3/1 -> SigConv_1/1
  Inport_3/1 -> RateTs_3/1

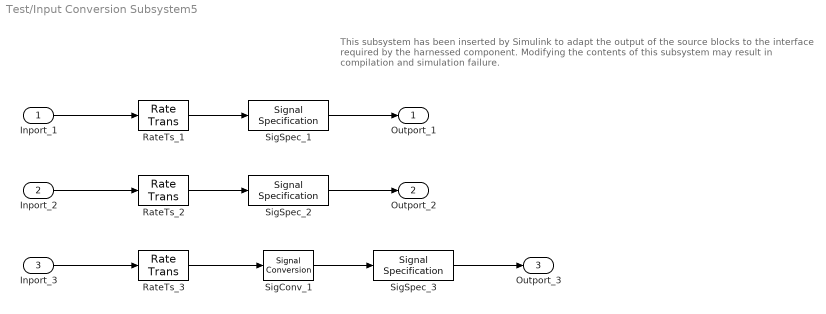
== system Test/Input Conversion Subsystem5 ==
  note: This subsystem has been inserted by Simulink to adapt the output of the source blocks to the interface required by the harnessed component.
      |  Modifying the contents of this subsystem may result in compilation and simulation failure.
  Inport_1 : Inport
  Inport_2 : Inport  Port=2
  Inport_3 : Inport  Port=3
  RateTs_1 : RateTransition  OutPortSampleTime=1
  RateTs_2 : RateTransition  OutPortSampleTime=1
  RateTs_3 : RateTransition  OutPortSampleTime=1
  SigConv_1 : SignalConversion  ConversionOutput=Virtual bus  OverrideOpt=off
  SigSpec_1 : SignalSpecification  OutDataTypeStr=boolean  Dimensions=[1]  SampleTime=1
  SigSpec_2 : SignalSpecification  OutDataTypeStr=boolean  Dimensions=[1]  SampleTime=1
  SigSpec_3 : SignalSpecification  OutDataTypeStr=Bus: fb_functions_out  SampleTime=1
  Outport_1 : Outport
  Outport_2 : Outport  Port=2
  Outport_3 : Outport  Port=3
  wires:
  SigSpec_1/1 -> Outport_1/1
  RateTs_1/1 -> SigSpec_1/1
  Inport_1/1 -> RateTs_1/1
  SigSpec_2/1 -> Outport_2/1
  RateTs_2/1 -> SigSpec_2/1
  Inport_2/1 -> RateTs_2/1
  SigSpec_3/1 -> Outport_3/1
  SigConv_1/1 -> SigSpec_3/1
  RateTs_3/1 -> SigConv_1/1
  Inport_3/1 -> RateTs_3/1

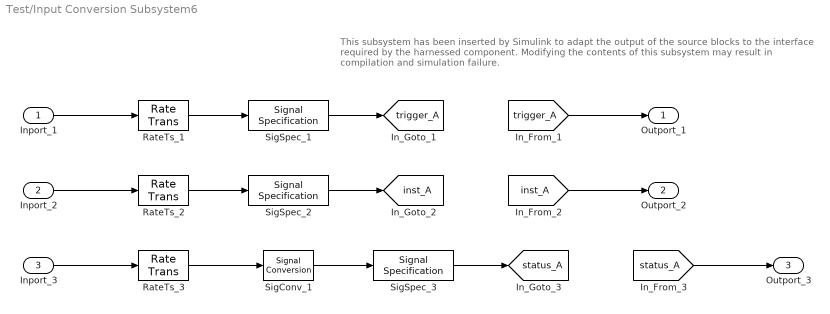
== system Test/Input Conversion Subsystem6 ==
  note: This subsystem has been inserted by Simulink to adapt the output of the source blocks to the interface required by the harnessed component.
      |  Modifying the contents of this subsystem may result in compilation and simulation failure.
  Inport_1 : Inport
  Inport_2 : Inport  Port=2
  Inport_3 : Inport  Port=3
  RateTs_1 : RateTransition  OutPortSampleTime=1
  RateTs_2 : RateTransition  OutPortSampleTime=1
  RateTs_3 : RateTransition  OutPortSampleTime=1
  SigConv_1 : SignalConversion  ConversionOutput=Virtual bus  OverrideOpt=off
  SigSpec_1 : SignalSpecification  OutDataTypeStr=boolean  Dimensions=[1]  SampleTime=1
  SigSpec_2 : SignalSpecification  OutDataTypeStr=int32  Dimensions=[1]  SampleTime=1
  SigSpec_3 : SignalSpecification  OutDataTypeStr=Bus: fb_status  SampleTime=1
  Outport_1 : Outport
  Outport_2 : Outport  Port=2
  Outport_3 : Outport  Port=3
  tag scope: inst_A=global, status_A=global, trigger_A=global
  wires:
  [trigger_A] -> Outport_1/1
  SigSpec_1/1 -> [trigger_A]
  RateTs_1/1 -> SigSpec_1/1
  Inport_1/1 -> RateTs_1/1
  [inst_A] -> Outport_2/1
  SigSpec_2/1 -> [inst_A]
  RateTs_2/1 -> SigSpec_2/1
  Inport_2/1 -> RateTs_2/1
  [status_A] -> Outport_3/1
  SigSpec_3/1 -> [status_A]
  SigConv_1/1 -> SigSpec_3/1
  RateTs_3/1 -> SigConv_1/1
  Inport_3/1 -> RateTs_3/1

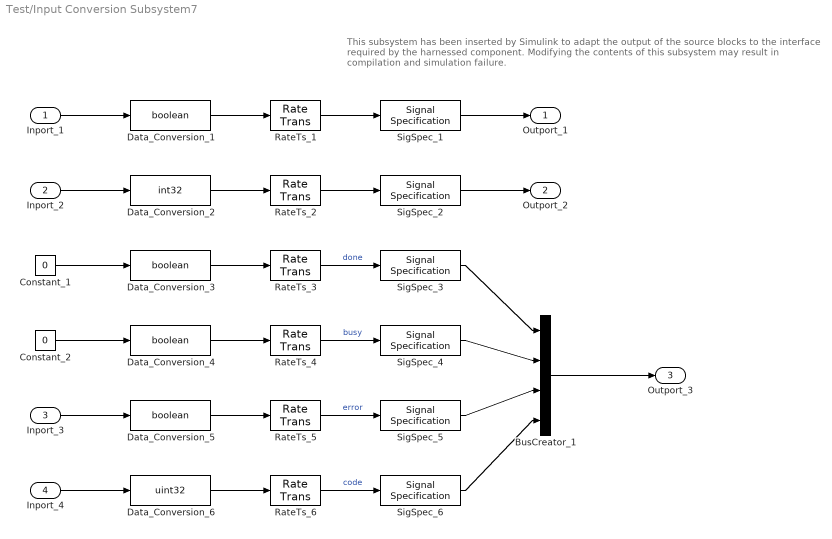
== system Test/Input Conversion Subsystem7 ==
  note: This subsystem has been inserted by Simulink to adapt the output of the source blocks to the interface required by the harnessed component.
      |  Modifying the contents of this subsystem may result in compilation and simulation failure.
  Inport_1 : Inport
  Inport_2 : Inport  Port=2
  Inport_3 : Inport  Port=3
  Inport_4 : Inport  Port=4
  BusCreator_1 : BusCreator  Inputs=4  OutDataTypeStr=Bus: fb_status
  Constant_1 : Constant  Value=0
  Constant_2 : Constant  Value=0
  Data_Conversion_{1,3..5} (4 alike) : DataTypeConversion  OutDataTypeStr=boolean  SaturateOnIntegerOverflow=on  RndMeth=Zero
  Data_Conversion_2 : DataTypeConversion  OutDataTypeStr=int32  SaturateOnIntegerOverflow=on  RndMeth=Zero
  Data_Conversion_6 : DataTypeConversion  OutDataTypeStr=uint32  SaturateOnIntegerOverflow=on  RndMeth=Zero
  RateTs_{1..6} (6 alike) : RateTransition  OutPortSampleTime=1
  SigSpec_{1,3..5} (4 alike) : SignalSpecification  OutDataTypeStr=boolean  Dimensions=[1]  SampleTime=1
  SigSpec_2 : SignalSpecification  OutDataTypeStr=int32  Dimensions=[1]  SampleTime=1
  SigSpec_6 : SignalSpecification  OutDataTypeStr=uint32  Dimensions=[1]  SampleTime=1
  Outport_1 : Outport
  Outport_2 : Outport  Port=2
  Outport_3 : Outport  Port=3
  wires:
  SigSpec_1/1 -> Outport_1/1
  RateTs_1/1 -> SigSpec_1/1
  Data_Conversion_1/1 -> RateTs_1/1
  Inport_1/1 -> Data_Conversion_1/1
  SigSpec_2/1 -> Outport_2/1
  RateTs_2/1 -> SigSpec_2/1
  Data_Conversion_2/1 -> RateTs_2/1
  Inport_2/1 -> Data_Conversion_2/1
  BusCreator_1/1 -> Outport_3/1
  SigSpec_3/1 -> BusCreator_1/1
  RateTs_3/1 -> SigSpec_3/1  "done"
  Data_Conversion_3/1 -> RateTs_3/1
  Constant_1/1 -> Data_Conversion_3/1
  SigSpec_4/1 -> BusCreator_1/2
  RateTs_4/1 -> SigSpec_4/1  "busy"
  Data_Conversion_4/1 -> RateTs_4/1
  Constant_2/1 -> Data_Conversion_4/1
  SigSpec_5/1 -> BusCreator_1/3
  RateTs_5/1 -> SigSpec_5/1  "error"
  Data_Conversion_5/1 -> RateTs_5/1
  Inport_3/1 -> Data_Conversion_5/1
  SigSpec_6/1 -> BusCreator_1/4
  RateTs_6/1 -> SigSpec_6/1  "code"
  Data_Conversion_6/1 -> RateTs_6/1
  Inport_4/1 -> Data_Conversion_6/1

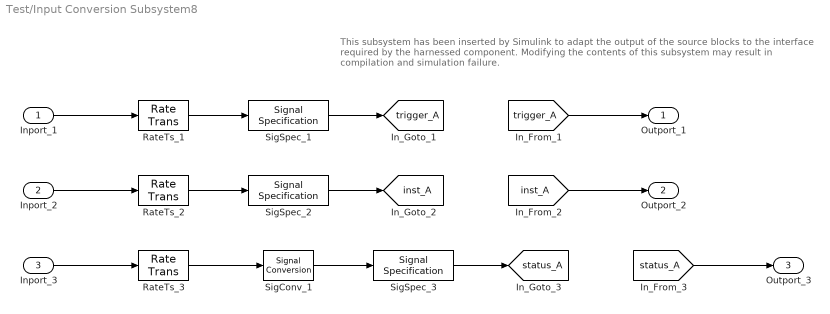
== system Test/Input Conversion Subsystem8 ==
  note: This subsystem has been inserted by Simulink to adapt the output of the source blocks to the interface required by the harnessed component.
      |  Modifying the contents of this subsystem may result in compilation and simulation failure.
  Inport_1 : Inport
  Inport_2 : Inport  Port=2
  Inport_3 : Inport  Port=3
  RateTs_1 : RateTransition  OutPortSampleTime=1
  RateTs_2 : RateTransition  OutPortSampleTime=1
  RateTs_3 : RateTransition  OutPortSampleTime=1
  SigConv_1 : SignalConversion  ConversionOutput=Virtual bus  OverrideOpt=off
  SigSpec_1 : SignalSpecification  OutDataTypeStr=boolean  Dimensions=[1]  SampleTime=1
  SigSpec_2 : SignalSpecification  OutDataTypeStr=int32  Dimensions=[1]  SampleTime=1
  SigSpec_3 : SignalSpecification  OutDataTypeStr=Bus: fb_status  SampleTime=1
  Outport_1 : Outport
  Outport_2 : Outport  Port=2
  Outport_3 : Outport  Port=3
  tag scope: inst_A=global, status_A=global, trigger_A=global
  wires:
  [trigger_A] -> Outport_1/1
  SigSpec_1/1 -> [trigger_A]
  RateTs_1/1 -> SigSpec_1/1
  Inport_1/1 -> RateTs_1/1
  [inst_A] -> Outport_2/1
  SigSpec_2/1 -> [inst_A]
  RateTs_2/1 -> SigSpec_2/1
  Inport_2/1 -> RateTs_2/1
  [status_A] -> Outport_3/1
  SigSpec_3/1 -> [status_A]
  SigConv_1/1 -> SigSpec_3/1
  RateTs_3/1 -> SigConv_1/1
  Inport_3/1 -> RateTs_3/1

== system Test/Output Conversion Subsystem ==
  note: This subsystem has been inserted by Simulink to adapt the output of the harnessed component to the interface required by the sink blocks.
      |  Modifying the contents of this subsystem may result in compilation and simulation failure.
  Inport_1 : Inport
  Outport_1 : Outport
  wires:
  Inport_1/1 -> Outport_1/1

== system Test/Output Conversion Subsystem1 ==
  note: This subsystem has been inserted by Simulink to adapt the output of the harnessed component to the interface required by the sink blocks.
      |  Modifying the contents of this subsystem may result in compilation and simulation failure.
  Inport_1 : Inport
  Outport_1 : Outport
  wires:
  Inport_1/1 -> Outport_1/1

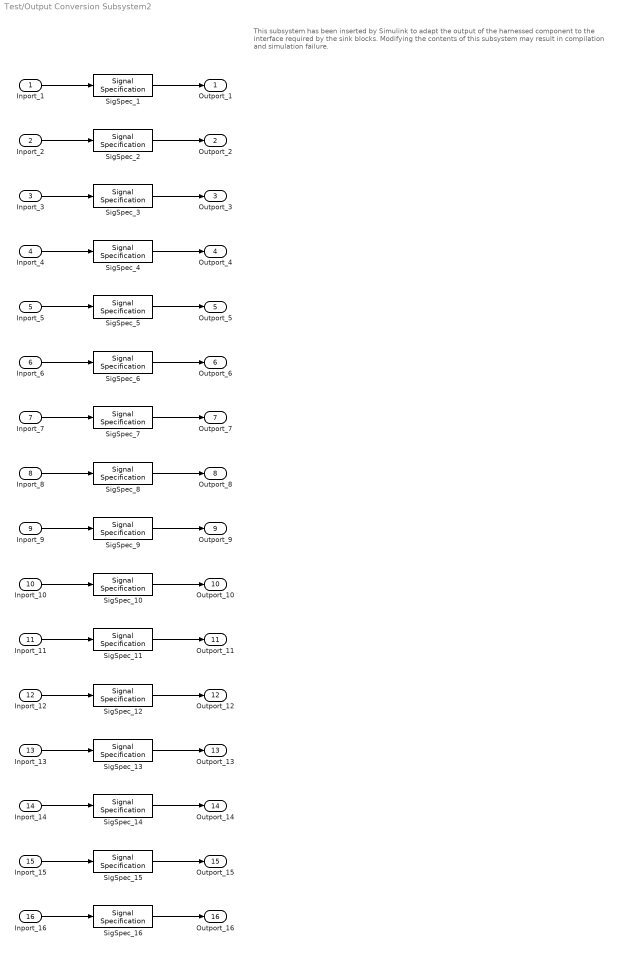
== system Test/Output Conversion Subsystem2 ==
  note: This subsystem has been inserted by Simulink to adapt the output of the harnessed component to the interface required by the sink blocks.
      |  Modifying the contents of this subsystem may result in compilation and simulation failure.
  Inport_1 : Inport
  Inport_2 : Inport  Port=2
  Inport_3 : Inport  Port=3
  Inport_4 : Inport  Port=4
  Inport_5 : Inport  Port=5
  Inport_6 : Inport  Port=6
  Inport_7 : Inport  Port=7
  Inport_8 : Inport  Port=8
  Inport_9 : Inport  Port=9
  Inport_10 : Inport  Port=10
  Inport_11 : Inport  Port=11
  Inport_12 : Inport  Port=12
  Inport_13 : Inport  Port=13
  Inport_14 : Inport  Port=14
  Inport_15 : Inport  Port=15
  Inport_16 : Inport  Port=16
  SigSpec_{1..2,5..7,10..16} (12 alike) : SignalSpecification  OutDataTypeStr=boolean  Dimensions=[1]  SampleTime=1
  SigSpec_3 : SignalSpecification  OutDataTypeStr=uint32  Dimensions=[1]  SampleTime=1
  SigSpec_4 : SignalSpecification  OutDataTypeStr=fixdt('ufix8_En1000')  Dimensions=[1]  SampleTime=1
  SigSpec_8 : SignalSpecification  OutDataTypeStr=uint8  Dimensions=[1]  SampleTime=1
  SigSpec_9 : SignalSpecification  OutDataTypeStr=Enum: StateFlowModeType  Dimensions=[1]  SampleTime=1
  Outport_1 : Outport
  Outport_2 : Outport  Port=2
  Outport_3 : Outport  Port=3
  Outport_4 : Outport  Port=4
  Outport_5 : Outport  Port=5
  Outport_6 : Outport  Port=6
  Outport_7 : Outport  Port=7
  Outport_8 : Outport  Port=8
  Outport_9 : Outport  Port=9
  Outport_10 : Outport  Port=10
  Outport_11 : Outport  Port=11
  Outport_12 : Outport  Port=12
  Outport_13 : Outport  Port=13
  Outport_14 : Outport  Port=14
  Outport_15 : Outport  Port=15
  Outport_16 : Outport  Port=16
  wires:
  Inport_1/1 -> SigSpec_1/1
  SigSpec_1/1 -> Outport_1/1
  Inport_2/1 -> SigSpec_2/1
  SigSpec_2/1 -> Outport_2/1
  Inport_3/1 -> SigSpec_3/1
  SigSpec_3/1 -> Outport_3/1
  Inport_4/1 -> SigSpec_4/1
  SigSpec_4/1 -> Outport_4/1
  Inport_5/1 -> SigSpec_5/1
  SigSpec_5/1 -> Outport_5/1
  Inport_6/1 -> SigSpec_6/1
  SigSpec_6/1 -> Outport_6/1
  Inport_7/1 -> SigSpec_7/1
  SigSpec_7/1 -> Outport_7/1
  Inport_8/1 -> SigSpec_8/1
  SigSpec_8/1 -> Outport_8/1
  Inport_9/1 -> SigSpec_9/1
  SigSpec_9/1 -> Outport_9/1
  Inport_10/1 -> SigSpec_10/1
  SigSpec_10/1 -> Outport_10/1
  Inport_11/1 -> SigSpec_11/1
  SigSpec_11/1 -> Outport_11/1
  Inport_12/1 -> SigSpec_12/1
  SigSpec_12/1 -> Outport_12/1
  Inport_13/1 -> SigSpec_13/1
  SigSpec_13/1 -> Outport_13/1
  Inport_14/1 -> SigSpec_14/1
  SigSpec_14/1 -> Outport_14/1
  Inport_15/1 -> SigSpec_15/1
  SigSpec_15/1 -> Outport_15/1
  Inport_16/1 -> SigSpec_16/1
  SigSpec_16/1 -> Outport_16/1
